simulink model "Controllore_Hinf"  (R2022b)
settings: Solver=ode113  StartTime=0.0  StopTime=10  RelTol=1e-3
values from neighbouring files (symbols this model uses):
  c1 = 6.54*10^(-2)    (= 0.0654)    [Progetto_CSI.m]
  c2 = 2.32*10^(-2)    (= 0.0232)    [Progetto_CSI.m]
  cond_iniz = [teta0(1);teta0(2);dteta0(1);dteta0(2)]    [Progetto_CSI.m]
  dteta0 = [0;0]    [Progetto_CSI.m]
  g = 9.81    [Progetto_CSI.m]
  I1 = 0.654    [Progetto_CSI.m]
  I2 = 0.117    [Progetto_CSI.m]
  Km1 = ureal('Km1',1.08,'Percentage',10)    [Progetto_CSI.m]
  Km2 = ureal('Km2',0.335,'Percentage',10)    [Progetto_CSI.m]
  Ktf = minreal(zpk(tf(K)))    [Progetto_CSI.m]
  l1 = 0.5    [Progetto_CSI.m]
  l2 = 0.4    [Progetto_CSI.m]
  M1 = 3.25    [Progetto_CSI.m]
  M2 = 1.90    (= 1.9)    [Progetto_CSI.m]
  Plant = minreal(ss(A,B,C,D))    [Progetto_CSI.m]
  teta0 = [0;0]    [Progetto_CSI.m]
  Tm1 = ureal('Tm1',0.005,'Percentage',20)    [Progetto_CSI.m]
  Tm2 = ureal('Tm2',0.002,'Percentage',20)    [Progetto_CSI.m]
  Wn = blkdiag(wn,wn)    [Progetto_CSI.m]
  Wp = blkdiag(wp,wp)    [Progetto_CSI.m]
  Wt = blkdiag(wt,wt)    [Progetto_CSI.m]
  Wu = blkdiag(wu,wu)    [Progetto_CSI.m]
undefined symbols (not defined in the file or in its folder): sigbuilder_block
settings Model: Creator=paoga  LastModifiedBy=paoga

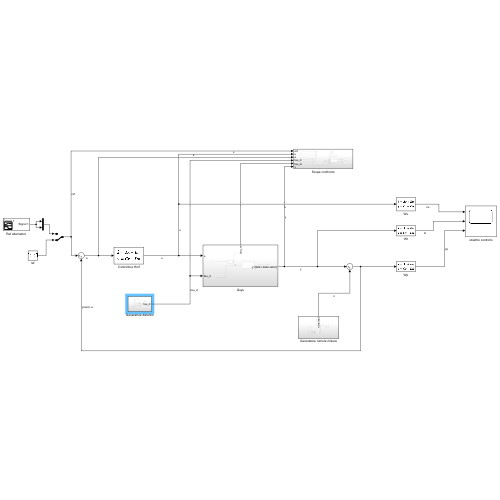
[thumbnail: Simulink's stored preview of the top-level diagram]
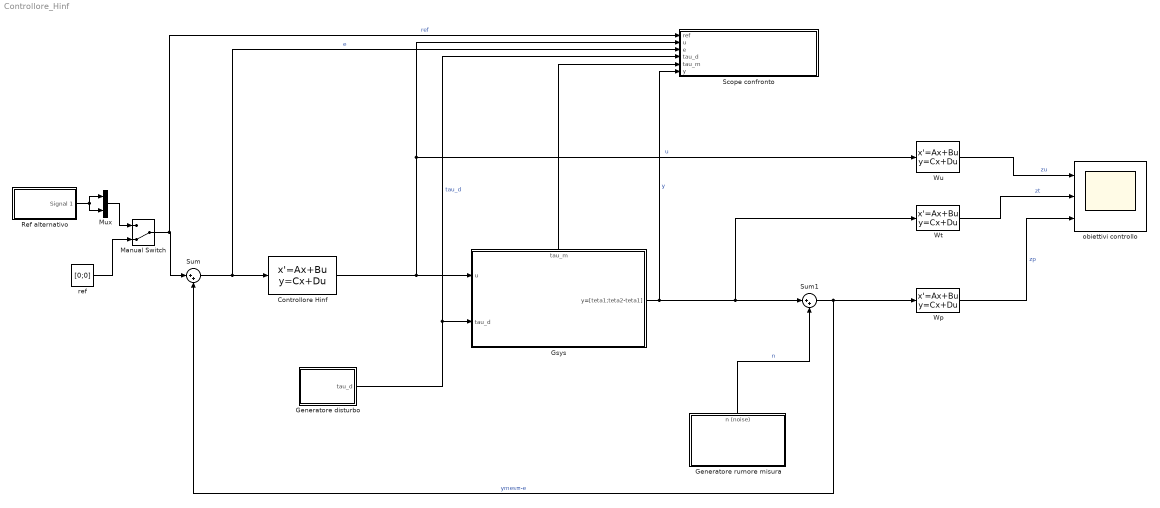
== system Controllore_Hinf ==
  Controllore Hinf : StateSpace  A=ss(Ktf,'min').A  B=ss(Ktf,'min').B  C=ss(Ktf,'min').C  D=ss(Ktf,'min').D  InitialCondition=0
  Generatore disturbo : Subsystem
  Generatore rumore misura : Subsystem
      settings: PortSchema="{\"entries\":[{\"content\":{\"sides\":[{\"content\":{\"connectorIds\":[]},\"type\":\"ConnectorPlacement.EquallySpacedRectSide\",\"uuid\":\"4563afe1-44c1-4b6e-ae92-57a13cb5f2ed\"},{\"content\":{\"connectorIds\":[],\"side\":\"RIGHT\"},\"type\":\"ConnectorPlacement.EquallySpacedRectSide\",\"uuid\":\"10cf2d49-a755-4040-b0d3-6221591ca79b\"},{\"content\":{\"connectorIds\":[\"Out1\"],\"side\":\"TOP\"},\"type\":\"ConnectorPlacement.EquallySpacedRectSide\",\"uuid\":\"737eed73-cf56-4396-8552-34a88d3a8214\"}]},\"type\":\"ConnectorPlacement.EquallySpacedConnector\",\"uuid\":\"4383ac91-74b1-450d-8a02-3f3d8ae1b6a0\"}],\"packageUris\":[\"http://schema.mathworks.com/mf0/Connector/R2020b\"],\"version\":\"1.0\"}"
  Gsys : Subsystem
      settings: PortSchema="{\"entries\":[{\"content\":{\"sides\":[{\"content\":{\"connectorIds\":[\"In1\",\"In2\"]},\"type\":\"ConnectorPlacement.EquallySpacedRectSide\",\"uuid\":\"18d893e1-8e34-4961-b34b-b4b9a69ed5ee\"},{\"content\":{\"connectorIds\":[\"Out1\"],\"side\":\"RIGHT\"},\"type\":\"ConnectorPlacement.EquallySpacedRectSide\",\"uuid\":\"8adab429-5027-4e99-8f69-c72e15093695\"},{\"content\":{\"connectorIds\":[\"Out2\"],\"side\":\"TOP\"},\"type\":\"ConnectorPlacement.EquallySpacedRectSide\",\"uuid\":\"82e68155-0a8a-4a9b-8dfc-7d42e2daa280\"}]},\"type\":\"ConnectorPlacement.EquallySpacedConnector\",\"uuid\":\"768b6bb2-d933-4015-ac22-1ce695ba2591\"}],\"packageUris\":[\"http://schema.mathworks.com/mf0/Connector/R2020b\"],\"version\":\"1.0\"}"
  Manual Switch : ManualSwitch  CurrentSetting=0
  Mux : Mux  Inputs=2
  Ref alternativo : Subsystem  Tag=STV Subsys  LoadFcn=sigbuilder_block('load');  StartFcn=sigbuilder_block('start');  StopFcn=sigbuilder_block('stop');  ClipboardFcn=sigbuilder_block('clipboard');  mask(Sigbuilder block){tuvar=[0:10]}
      mask help: Simulink:masks:SigbuilderBlock_MD
      mask init:
      | if ~strcmp(get_param(bdroot(gcbh),'SimulationStatus'),'stopped') tuvar = sigbuilder_block('maskInit'); end
      settings: CopyFcn=sigbuilder_block('copy');  DeleteFcn=sigbuilder_block('delete');  ModelCloseFcn=sigbuilder_block('modelClose');  PreSaveFcn=sigbuilder_block('preSave');  PauseFcn=sigbuilder_block('pause');  ContinueFcn=sigbuilder_block('continue');  NameChangeFcn=sigbuilder_block('namechange');  OpenFcn=sigbuilder_block('open',[5.4 36 1141.2 516.6 ]);  CloseFcn=sigbuilder_block('close');
      mask Display: plot(0, 0, 100, 100,[2, 2, 32, 32, 2], [68, 8, 8, 68, 68],[32, 2], [38, 38], [32, 19, 2],[53, 60, 44], [32, 17, 17, 2],[16, 16, 31, 31]);txt = getActiveGroup(gcbh);text(2, 100, txt,'verticalAlignment', 'top');
  Scope confronto : Subsystem
  Sum : Sum  Inputs=|++
  Sum1 : Sum  Inputs=|++
  Wp : StateSpace  A=ss(Wp,'min').A  B=ss(Wp,'min').B  C=ss(Wp,'min').C  D=ss(Wp,'min').D  InitialCondition=0
  Wt : StateSpace  A=ss(Wt,'min').A  B=ss(Wt,'min').B  C=ss(Wt,'min').C  D=ss(Wt,'min').D  InitialCondition=0
  Wu : StateSpace  A=ss(Wu,'min').A  B=ss(Wu,'min').B  C=ss(Wu,'min').C  D=ss(Wu,'min').D  InitialCondition=0
  obiettivi controllo : Scope  NumInputPorts=3
  ref : Constant  Value=[0;0]
  wires:
  Controllore Hinf/1 -> Wu/1, Scope confronto/2(u), Gsys/1(u)  "u"
  Gsys/1(y=[teta1;teta2-teta1]) -> Scope confronto/6(y), Wt/1, Sum1/1  "y"
  ref/1 -> Manual Switch/2
  Generatore rumore misura/1(n (noise)) -> Sum1/2  "n"
  Sum1/1 -> Wp/1, Sum/2  "ymes=-e"
  Wp/1 -> obiettivi controllo/3  "zp"
  Wt/1 -> obiettivi controllo/2  "zt"
  Wu/1 -> obiettivi controllo/1  "zu"
  Sum/1 -> Scope confronto/3(e), Controllore Hinf/1  "e"
  Gsys/2(tau_m) -> Scope confronto/5(tau_m)
  Generatore disturbo/1(tau_d) -> Scope confronto/4(tau_d), Gsys/2(tau_d)  "tau_d"
  Ref alternativo/1(Signal 1) -> Mux/2, Mux/1
  Mux/1 -> Manual Switch/1
  Manual Switch/1 -> Scope confronto/1(ref), Sum/1  "ref"

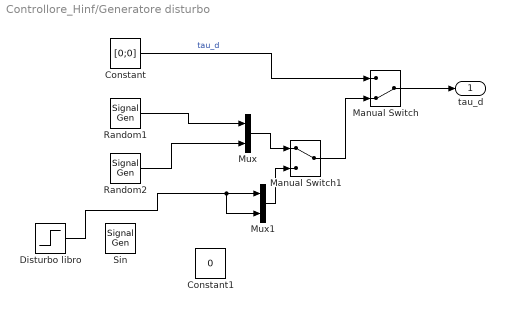
== system Controllore_Hinf/Generatore disturbo ==
  Constant : Constant  Value=[0;0]
  Constant1 : Constant  Value=0
  Disturbo libro : Step  After=0.1  SampleTime=0
  Manual Switch : ManualSwitch  CurrentSetting=0
  Manual Switch1 : ManualSwitch
  Mux : Mux  Inputs=2
  Mux1 : Mux  Inputs=2
  Random1 : SignalGenerator  WaveForm=random  Amplitude=100  Units=rad/sec
  Random2 : SignalGenerator  WaveForm=random  Amplitude=100  Units=rad/sec
  Sin : SignalGenerator  Amplitude=100  Frequency=0.5  Units=rad/sec
  tau_d : Outport
  wires:
  Mux/1 -> Manual Switch1/1
  Constant/1 -> Manual Switch/1  "tau_d"
  Manual Switch/1 -> tau_d/1
  Random1/1 -> Mux/1
  Random2/1 -> Mux/2
  Manual Switch1/1 -> Manual Switch/2
  Mux1/1 -> Manual Switch1/2
  Disturbo libro/1 -> Mux1/2, Mux1/1

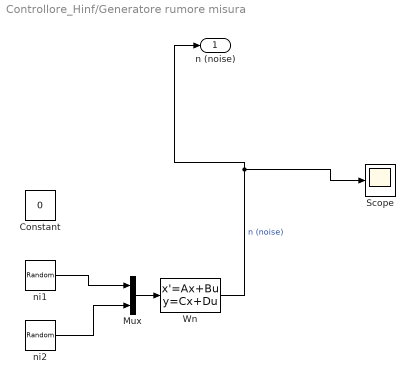
== system Controllore_Hinf/Generatore rumore misura ==
  Constant : Constant  Value=0
  Mux : Mux  Inputs=2
  Scope : Scope
  Wn : StateSpace  A=ss(Wn).A  B=ss(Wn).B  C=ss(Wn).C  D=ss(Wn).D  InitialCondition=0
  ni1 : RandomNumber  Variance=0.03^2  SampleTime=0.1
  ni2 : RandomNumber  Variance=0.03^2  SampleTime=0.1
  n (noise) : Outport
  wires:
  Mux/1 -> Wn/1
  Wn/1 -> Scope/1, n (noise)/1  "n (noise)"
  ni1/1 -> Mux/1
  ni2/1 -> Mux/2

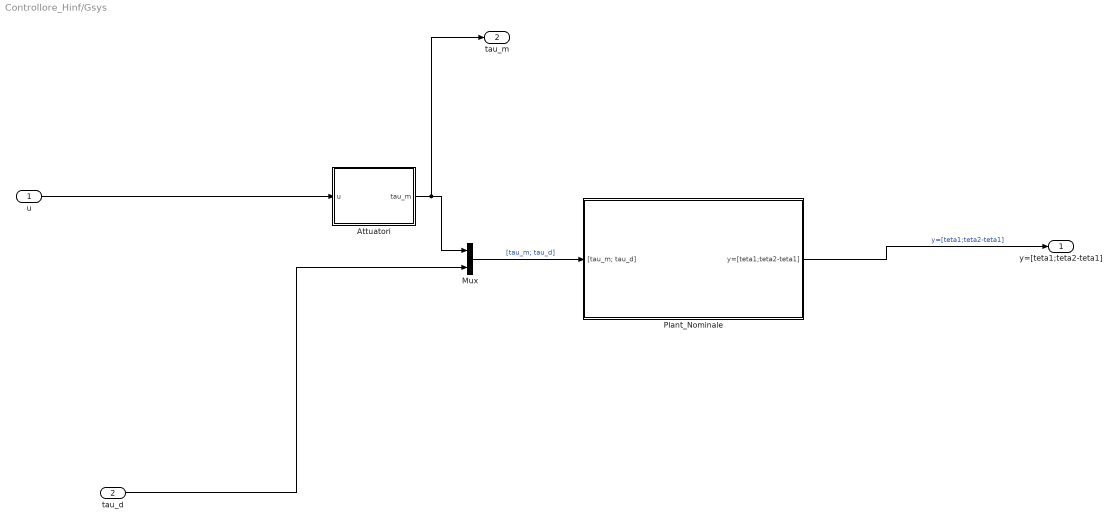
== system Controllore_Hinf/Gsys ==
  u : Inport
  tau_d : Inport  Port=2
  Attuatori : Subsystem
  Mux : Mux  Inputs=2
  Plant_Nominale : Subsystem
  y=[teta1;teta2-teta1] : Outport
  tau_m : Outport  Port=2
  wires:
  tau_d/1 -> Mux/2
  u/1 -> Attuatori/1(u)
  Attuatori/1(tau_m) -> tau_m/1, Mux/1
  Plant_Nominale/1(y=[teta1;teta2-teta1]) -> y=[teta1;teta2-teta1]/1  "y=[teta1;teta2-teta1]"
  Mux/1 -> Plant_Nominale/1("[tau_m; tau_d]")  "[tau_m; tau_d]"

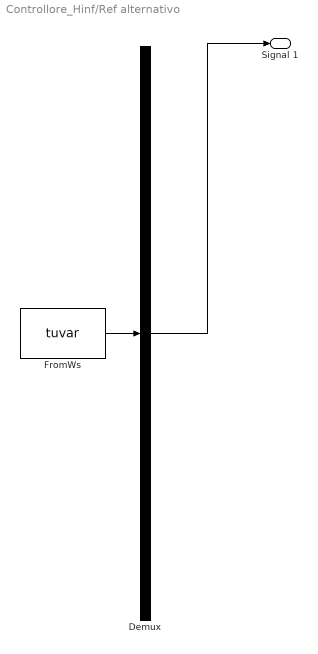
== system Controllore_Hinf/Ref alternativo ==
  Demux : Demux  Tag=STV Demux  Outputs=1
      settings: DisplayOption=none
  FromWs : FromWorkspace  Tag=STV FromWs  VariableName=tuvar
      SigBuilderData=|
      | common.afterFinalStr = 'Extrapolate'
      | common.sampleTime = 0
      | dataSet.timeRange = [0 10]
      | dataSet.name = 'Group 1'
      | sbobj.Groups.Name = 'Group 1'
      | sbobj.Groups.Signals.Name = 'Signal 1'
      | sbobj.Groups.Signals.XData = [0 4 4.1 4.22 4.35 4.5 4.75 7 7.25 7.5 7.55 7.75 8 10]
      | sbobj.Groups.Signals.YData = [0 0 0.15 1.01 1.16 1.31 1.36 1.37 1.32 1.15 0.98 0.18 0 0]
  Signal 1 : Outport  Tag=STV Outport
  wires:
  Demux/1 -> Signal 1/1
  FromWs/1 -> Demux/1

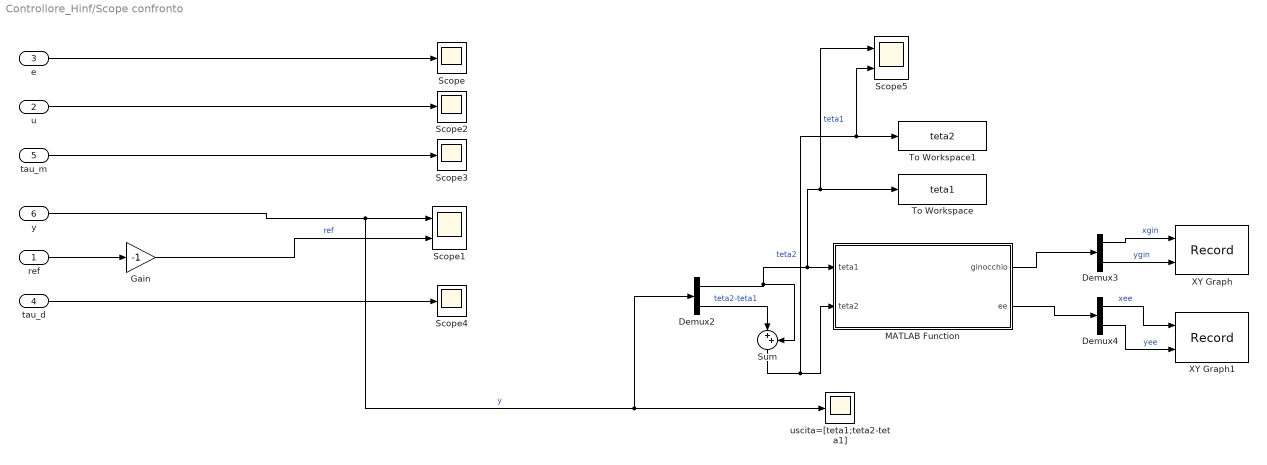
== system Controllore_Hinf/Scope confronto ==
  ref : Inport
  u : Inport  Port=2
  e : Inport  Port=3
  tau_d : Inport  Port=4
  tau_m : Inport  Port=5
  y : Inport  Port=6
  Demux2 : Demux  Outputs=2
  Demux3 : Demux  Outputs=2
  Demux4 : Demux  Outputs=2
  Gain : Gain  Gain=-1
  MATLAB Function : MATLAB Function  TreatAsAtomicUnit=on
  Scope{,2..4} (4 alike) : Scope
  Scope1 : Scope  NumInputPorts=2
  Scope5 : Scope  NumInputPorts=2
  Sum : Sum  Inputs=|++
  To Workspace : ToWorkspace  VariableName=teta1  SaveFormat=Timeseries  SampleTime=0.001
  To Workspace1 : ToWorkspace  VariableName=teta2  SaveFormat=Timeseries  SampleTime=0.001
  XY Graph : Record  FileSettingsInternal="{\"entries\":[{\"content\":{\"excelSettings\":{\"content\":{},\"type\":\"Streamout.ExcelSettings\"}},\"type\":\"Streamout.FileSettingStorage\",\"uuid\":\"d28b810d-8f5e-49bf-8304-745c967aae85\"}],\"packageUris\":[\"http://schema.mathworks.com/mf0/streamout_blocks/R2020a\"],\"version\":\"1.0\"}"  Layout=[1 1]  SignalsInternal="{\"entries\":[{\"content\":{\"signals\":[{\"content\":{\"blockPath\":[\"Controllore_Hinf/Scope confronto/XY Graph\"],\"channel\":[],\"dimensions\":[1,1],\"domain\":\"Controllore_Hinf/Scope confronto/XY Graph\",\"lineColor\":\"#edb120\",\"plots\":[1],\"port\":1,\"sid\":[\"\"],\"signalID\":3957,\"signalName\":\"xgin\"},\"type\":\"RecordBlkView.Signal\",\"uuid\":\"8076e5f7-8ed5-48cf-9b82-05484cb4dd0f\"},{\"content\":{\"blockPath\":[\"Controllore_Hinf/Scope confronto/XY Graph\"],\"channel\":[],\"dimensions\":[1,1],\"domain\":\"Controllore_Hinf/Scope confronto/XY Graph\",\"lineColor\":\"#139fff\",\"plots\":[1],\"port\":2,\"sid\":[\"\"],\"signalID\":3961,\"signalName\":\"ygin\"},\"type\":\"RecordBlkView.Signal\",\"uuid\":\"f23da77b-08bc-4437-a0ff-a8dce06db6d0\"}]},\"type\":\"RecordBlkView.InputSignals\",\"uuid\":\"25ff8908-8420-489c-b6be-febb83001814\"}],\"packageUris\":[\"http://schema.mathworks.com/mf0/streamout_blocks/R2020a\"],\"version\":\"1.0\"}"  VisualizationBindings="{\"sparklinesplugin\":{\"info\":[{\"bindingParametersList\":[],\"subplotID\":1}]}}"  CompatibilityTag=XY
  XY Graph1 : Record  FileSettingsInternal="{\"entries\":[{\"content\":{\"excelSettings\":{\"content\":{},\"type\":\"Streamout.ExcelSettings\"}},\"type\":\"Streamout.FileSettingStorage\",\"uuid\":\"866a8769-9de0-469a-acad-6cec99dd1763\"}],\"packageUris\":[\"http://schema.mathworks.com/mf0/streamout_blocks/R2020a\"],\"version\":\"1.0\"}"  Layout=[1 1]  SignalsInternal="{\"entries\":[{\"content\":{\"signals\":[{\"content\":{\"blockPath\":[\"Controllore_Hinf/Scope confronto/XY Graph1\"],\"channel\":[],\"dimensions\":[1,1],\"domain\":\"Controllore_Hinf/Scope confronto/XY Graph1\",\"lineColor\":\"#77ac30\",\"plots\":[1],\"port\":1,\"sid\":[\"\"],\"signalID\":3965,\"signalName\":\"xee\"},\"type\":\"RecordBlkView.Signal\",\"uuid\":\"24aef917-77c4-4924-9836-a8d9a3bdd47d\"},{\"content\":{\"blockPath\":[\"Controllore_Hinf/Scope confronto/XY Graph1\"],\"channel\":[],\"dimensions\":[1,1],\"domain\":\"Controllore_Hinf/Scope confronto/XY Graph1\",\"lineColor\":\"#64d413\",\"plots\":[1],\"port\":2,\"sid\":[\"\"],\"signalID\":3969,\"signalName\":\"yee\"},\"type\":\"RecordBlkView.Signal\",\"uuid\":\"0ad6965d-abf5-4901-a9ed-38c6eab061da\"}]},\"type\":\"RecordBlkView.InputSignals\",\"uuid\":\"73f47fe2-fa1e-4cd6-9d34-c2b9358e14b4\"}],\"packageUris\":[\"http://schema.mathworks.com/mf0/streamout_blocks/R2020a\"],\"version\":\"1.0\"}"  VisualizationBindings="{\"sparklinesplugin\":{\"info\":[{\"bindingParametersList\":[],\"subplotID\":1}]}}"  CompatibilityTag=XY
  uscita=[teta1;teta2-teta1] : Scope
  wires:
  e/1 -> Scope/1
  u/1 -> Scope2/1
  tau_m/1 -> Scope3/1
  tau_d/1 -> Scope4/1
  ref/1 -> Gain/1
  Gain/1 -> Scope1/2  "ref"
  Demux4/1 -> XY Graph1/1  "xee"
  Demux3/2 -> XY Graph/2  "ygin"
  Demux3/1 -> XY Graph/1  "xgin"
  MATLAB Function/1(ginocchio) -> Demux3/1
  Demux2/1 -> Scope5/1, To Workspace/1, MATLAB Function/1(teta1), Sum/2  "teta1"
  Sum/1 -> Scope5/2, To Workspace1/1, MATLAB Function/2(teta2)  "teta2"
  Demux4/2 -> XY Graph1/2  "yee"
  MATLAB Function/2(ee) -> Demux4/1
  y/1 -> uscita=[teta1;teta2-teta1]/1, Demux2/1, Scope1/1  "y"
  Demux2/2 -> Sum/1  "teta2-teta1"

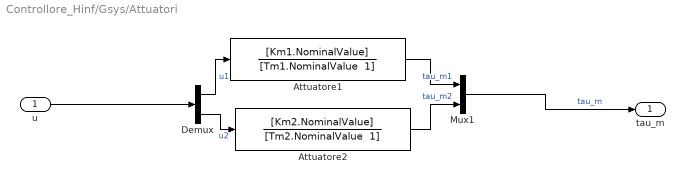
== system Controllore_Hinf/Gsys/Attuatori ==
  u : Inport
  Attuatore1 : TransferFcn  Numerator=[Km1.NominalValue]  Denominator="[Tm1.NominalValue  1]"
  Attuatore2 : TransferFcn  Numerator=[Km2.NominalValue]  Denominator="[Tm2.NominalValue  1]"
  Demux : Demux  Outputs=2
  Mux1 : Mux  Inputs=2
  tau_m : Outport
  wires:
  Attuatore2/1 -> Mux1/2  "tau_m2"
  Mux1/1 -> tau_m/1  "tau_m"
  Demux/1 -> Attuatore1/1  "u1"
  Attuatore1/1 -> Mux1/1  "tau_m1"
  Demux/2 -> Attuatore2/1  "u2"
  u/1 -> Demux/1

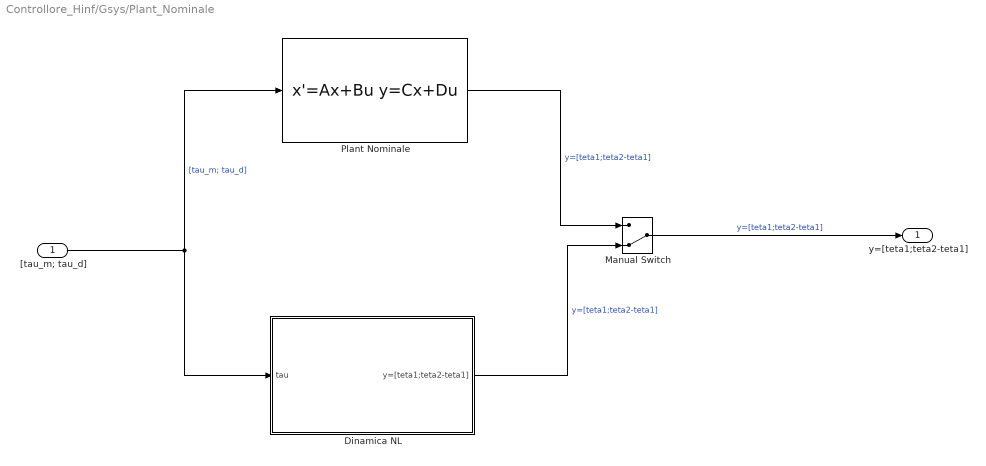
== system Controllore_Hinf/Gsys/Plant_Nominale ==
  "[tau_m; tau_d]" : Inport
  Dinamica NL : Subsystem
  Manual Switch : ManualSwitch  CurrentSetting=0
  Plant Nominale : StateSpace  A=Plant.NominalValue.A  B=Plant.NominalValue.B  C=Plant.NominalValue.C  D=Plant.NominalValue.D  InitialCondition=cond_iniz
  y=[teta1;teta2-teta1] : Outport
  wires:
  Plant Nominale/1 -> Manual Switch/1  "y=[teta1;teta2-teta1]"
  "[tau_m; tau_d]"/1 -> Dinamica NL/1(tau), Plant Nominale/1  "[tau_m; tau_d]"
  Manual Switch/1 -> y=[teta1;teta2-teta1]/1  "y=[teta1;teta2-teta1]"
  Dinamica NL/1(y=[teta1;teta2-teta1]) -> Manual Switch/2  "y=[teta1;teta2-teta1]"

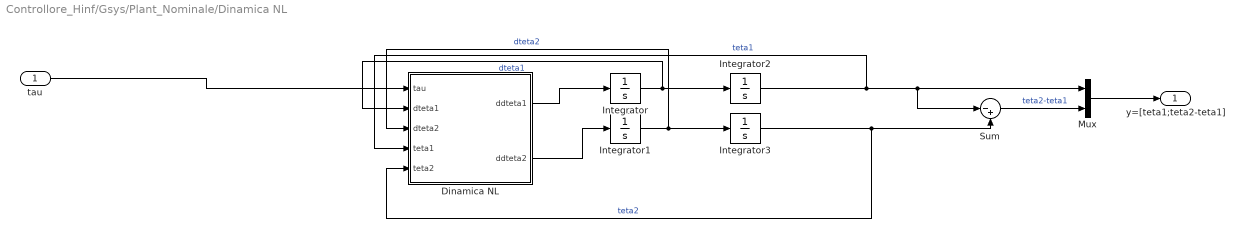
== system Controllore_Hinf/Gsys/Plant_Nominale/Dinamica NL ==
  tau : Inport
  Dinamica NL : MATLAB Function  TreatAsAtomicUnit=on
  Integrator : Integrator  InitialCondition=dteta0(1)
  Integrator1 : Integrator  InitialCondition=dteta0(2)
  Integrator2 : Integrator  InitialCondition=teta0(1)
  Integrator3 : Integrator  InitialCondition=teta0(2)
  Mux : Mux  Inputs=2
  Sum : Sum  Inputs=|-+
  y=[teta1;teta2-teta1] : Outport
  wires:
  Dinamica NL/1(ddteta1) -> Integrator/1
  Dinamica NL/2(ddteta2) -> Integrator1/1
  tau/1 -> Dinamica NL/1(tau)
  Integrator/1 -> Dinamica NL/2(dteta1), Integrator2/1  "dteta1"
  Integrator1/1 -> Dinamica NL/3(dteta2), Integrator3/1  "dteta2"
  Integrator2/1 -> Sum/1, Mux/1, Dinamica NL/4(teta1)  "teta1"
  Integrator3/1 -> Dinamica NL/5(teta2), Sum/2  "teta2"
  Sum/1 -> Mux/2  "teta2-teta1"
  Mux/1 -> y=[teta1;teta2-teta1]/1

== matlab function Controllore_Hinf/Scope confronto/MATLAB Function ==
  data: teta1 input; ginocchio output; teta2 input; ee output
function [ginocchio,ee] = fcn(teta1,teta2)
l1=0.5;l2=0.4;
ginocchio=[l1*sin(teta1);
           l1*cos(teta1)];
ee=ginocchio+[l2*sin(teta2);
           l2*cos(teta2)];
end

== matlab function Controllore_Hinf/Gsys/Plant_Nominale/Dinamica NL/Dinamica NL ==
  data: tau input; ddteta1 output; dteta1 input; ddteta2 output; dteta2 input; teta1 input; teta2 input; I1 parameter; I2 parameter; M1 parameter; M2 parameter; l1 parameter; l2 parameter; c1 parameter; c2 parameter; g parameter
function [ddteta1,ddteta2]=dinamicaNL(tau,dteta1,dteta2,teta1,teta2,I1, I2, M1, M2, l1, l2, c1, c2, g)
h1nom=0.35;
h2nom=0.181;
tau_m=tau(1:2);tau_d=tau(3:4);
dteta=[dteta1;dteta2];
M=[I1+M1*h1nom^2+M2*l1^2  l1*M2*cos(teta1-teta2);
    l1*M2*cos(teta1-teta2)  I2+M2*h2nom^2];
N=[c1+c2  -c2;
    -c2  c2];
q=[l1*M2*sin(teta1-teta2)*dteta2^2-M1*g*sin(teta1)
    l1*M2*sin(teta1-teta2)*dteta1^2-M2*g*sin(teta2)];
G=[1 0;
    -1 1];
T=[1 -1;
    0 1];
ddteta=pinv(M)*(G*tau_m+T*tau_d-N*dteta-q);
ddteta1=ddteta(1);
ddteta2=ddteta(2);
end
